simulink library "myLibrary"  (R2017b)
settings: Solver=VariableStepAuto  StartTime=0.0  StopTime=10.0  RelTol=1e-3
undefined symbols (not defined in the file): p, windData
libraries: aerolibwind2 x7, lowLevel x4, myLibrary x3, simulink x2, aerolibwindfilters x1, sharedtransform x1
settings Model: Creator=M.Cobb  LastModifiedBy=M.Cobb
settings CodeAppCC: StateflowObjectComments=on

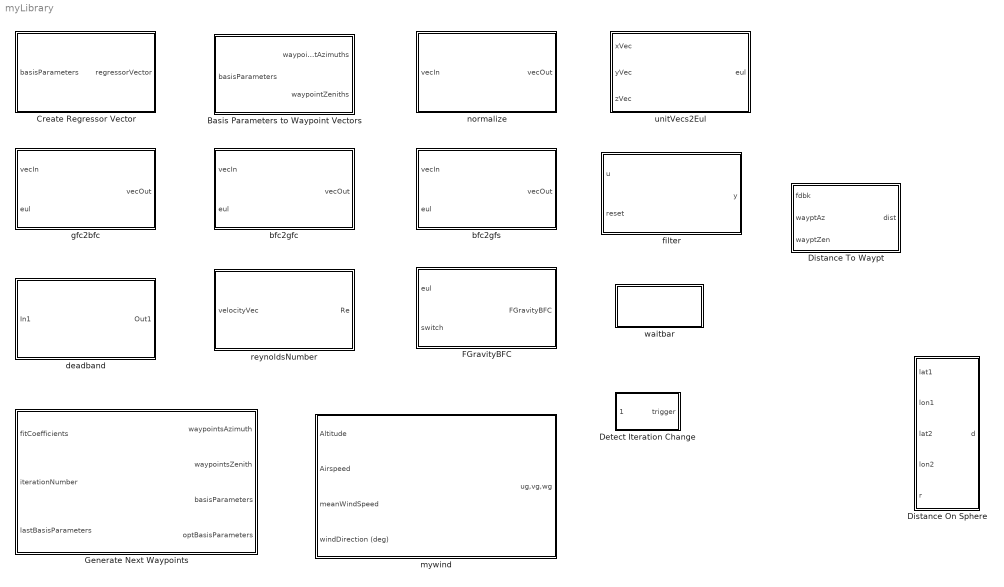
== system myLibrary ==
  Basis Parameters to Waypoint Vectors : Subsystem
  Create Regressor Vector : Subsystem
  Detect Iteration Change : Subsystem
  Distance On Sphere : Subsystem
  Distance To Waypt : Subsystem
  FGravityBFC : Subsystem
  Generate Next Waypoints : Subsystem
  bfc2gfc : Subsystem
  bfc2gfs : Subsystem
  deadband : Subsystem
  filter : Subsystem
  gfc2bfc : Subsystem
  mywind : Subsystem  mask(Wind Turbulence Model){units=Metric (MKS), spec=MIL-F-8785C, model=Continuous Von Karman (+q +r), Wdeg=0, TurbProb=10^-2 - Light, L_high=762, Wingspan=p.wingSpan, ts=p.Ts, Seed=[23341 23342 23343 23344], T_on=on}
      mask prompts: units "aeroblks:aeroblkwind:blockWindTurbulenceModelParamUnits"; spec "aeroblks:aeroblkwind:blockWindTurbulenceModelParamSpecification"; model "aeroblks:aeroblkwind:blockWindTurbulenceModelParamModeltype"; Wdeg "Wind direction at 6 m (degrees clockwise from north):"; TurbProb "aeroblks:aeroblkwind:blockWindTurbulenceModelParamProbabilityofexceedanceofhighaltitudeintensity"; L_high "Scale length at medium/high altitudes (m):"; Wingspan "Wingspan (m):"; ts "Band limited noise sample time (sec):"; Seed "Band limited noise sample time (sec):"; T_on "aeroblks:aeroblkwind:blockWindTurbulenceModelParamTurbulenceon"
      mask help: aeroblks:aeroblkwind:blockWindTurbulenceModelDesc
      mask init:
      | % index = strfind(model,' ');
      | % disp1 = model(1:index(1)-1);
      | % disp2 = model(index(1)+1:index(end-1)-1);
      | % disp3 = model(index(end-1)+1:end);
      | % 
      | h_vec = [.5 1.75 3.75 7.5 15 25 35 45 55 65 75 80]*1000;% feet
      | sigma_vec(1,:) = [3.2 2.2 1.5 zeros(1,9)]; % ft/sec
      | sigma_vec(2,:) = [4.2 3.6 3.3 1.6 zeros(1,8)];
      | sigma_vec(3,:) = [6.6 6.9 7.4 6.7 4.6 2.7 0.4 zeros(1,5)];
      | sigma_vec(4,:) = [8.6 9.6 10.6 10.1 8.0 6.6 5.0 4.2 2.7 zeros(1,3)];
      | sigma_vec(5,:) = [11.8 13.0 16.0 15.1 11.6 9.7 8.1 8.2 7.9 4.9 3.2 2.1];
      | sigma_vec(6,:) = [15.6 17.6 23.0 23.6 22.1 20.0 16.0 15.1 12.1 7.9 6.2 5.1];
      | sigma_vec(7,:) = [18.7 21.5 28.4 30.2 30.7 31.0 25.2 23.1 17.5 10.7 8.4 7.2];
      | max_height_low = 1000;
      | if strcmp(spec,'MIL-F-8785C')
      |     min_height_high = 2000;
      | else
      | 	min_height_high = 1750;
      | end
      | % [ports] = aeroicon('aeroblkwindturb2','icon');
      | % 
      | % dt=ts;
      mask Help: eval('asbhelp(''Von Karman Wind Turbulence Model (Continuous)'')');
      mask TypeOptions units: aeroblks:aeroblkwind:blockWindTurbulenceModelParamComboMetricMKS | aeroblks:aeroblkwind:blockWindTurbulenceModelParamComboEnglishVelocityinfts | aeroblks:aeroblkwind:blockWindTurbulenceModelParamComboEnglishVelocityinkts
      mask TypeOptions spec: aeroblks:aeroblkwind:blockWindTurbulenceModelParamComboMILF8785C | aeroblks:aeroblkwind:blockWindTurbulenceModelParamComboMILHDBK1797 | aeroblks:aeroblkwind:blockWindTurbulenceModelParamComboMILHDBK1797B
      mask TypeOptions model: aeroblks:aeroblkwind:blockWindTurbulenceModelParamComboContinuousVonKarmanqr1 | aeroblks:aeroblkwind:blockWindTurbulenceModelParamComboContinuousVonKarmanqr2 | aeroblks:aeroblkwind:blockWindTurbulenceModelParamComboContinuousVonKarmanqr3 | aeroblks:aeroblkwind:blockWindTurbulenceModelParamComboContinuousDrydenqr1 | aeroblks:aeroblkwind:blockWindTurbulenceModelParamComboContinuousDrydenqr2 | aeroblks:aeroblkwind:blockWindTurbulenceModelParamComboContinuousDrydenqr3 | aeroblks:aeroblkwind:blockWindTurbulenceModelParamComboDiscreteDrydenqr1 | aeroblks:aeroblkwind:blockWindTurbulenceModelParamComboDiscreteDrydenqr2 | aeroblks:aeroblkwind:blockWindTurbulenceModelParamComboDiscreteDrydenqr3
      mask Callback model: aeroicon('aeroblkwindturb2');
      mask TypeOptions TurbProb: aeroblks:aeroblkwind:blockWindTurbulenceModelParamCombo2x101 | aeroblks:aeroblkwind:blockWindTurbulenceModelParamCombo101 | aeroblks:aeroblkwind:blockWindTurbulenceModelParamCombo102Light | aeroblks:aeroblkwind:blockWindTurbulenceModelParamCombo103Moderate | aeroblks:aeroblkwind:blockWindTurbulenceModelParamCombo104 | aeroblks:aeroblkwind:blockWindTurbulenceModelParamCombo105Severe | aeroblks:aeroblkwind:blockWindTurbulenceModelParamCombo106
      mask Display:
      | port_label('output',1,'vWind','texmode','on');
      | port_label('input',1,'altitude (m)','texmode','on');
      | port_label('input',2,'airspeed (m/s)','texmode','on');
      | port_label('input',3,'meanWindSpeed (m/s)','texmode','on');
      | port_label('input',4,'wind direction (deg)','texmode','on');
      | % port_label(ports(5).type,ports(5).port,ports(5).txt,'texmode','on');
      | % [x y highstr lowstr maxy miny] = aeroimage('wind',gcbh,[disp2 '\n' disp3],disp1);
      | % plot(x,y)
      | % text(0.5,miny-0.05,lowstr,'HorizontalAlignment','center','verticalalignment','top')
      | % text(0.5,maxy,highstr,'HorizontalAlignment','center','verticalalignment','bottom')
  normalize : Subsystem
  reynoldsNumber : Subsystem
  unitVecs2Eul : Subsystem
  waitbar : Subsystem

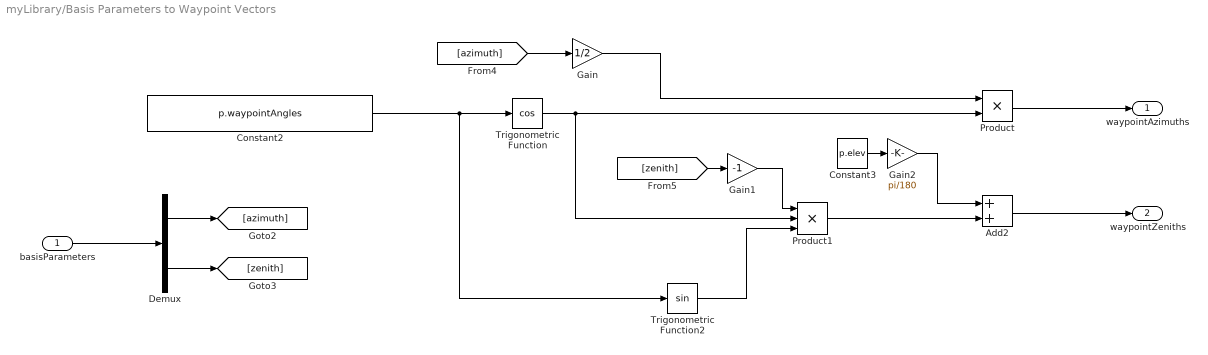
== system myLibrary/Basis Parameters to Waypoint Vectors ==
  basisParameters : Inport
  Add2 : Sum
  Constant2 : Constant  Value=p.waypointAngles  SampleTime=-1
  Constant3 : Constant  Value=p.elev
  Demux : Demux  Outputs=2
  Gain : Gain  Gain=1/2
  Gain1 : Gain  Gain=-1
  Gain2 : Gain  Gain=pi/180
  Product : Product
  Product1 : Product  Inputs=3
  Trigonometric Function : Trigonometry  Operator=cos
  Trigonometric Function2 : Trigonometry
  waypointAzimuths : Outport
  waypointZeniths : Outport  Port=2
  wires:
  Gain/1 -> Product/1
  Product1/1 -> Add2/2
  Trigonometric Function2/1 -> Product1/3
  [azimuth] -> Gain/1
  Constant2/1 -> Trigonometric Function2/1, Trigonometric Function/1
  basisParameters/1 -> Demux/1
  Demux/1 -> [azimuth]
  [zenith] -> Gain1/1
  Gain1/1 -> Product1/1
  Demux/2 -> [zenith]
  Trigonometric Function/1 -> Product1/2, Product/2
  Constant3/1 -> Gain2/1
  Product/1 -> waypointAzimuths/1
  Add2/1 -> waypointZeniths/1
  Gain2/1 -> Add2/1

== system myLibrary/Create Regressor Vector ==
  basisParameters : Inport  PortDimensions=2
  Constant2 : Constant
  Demux : Demux  Outputs=2
  Mux : Mux  Inputs=5
  Product : Product
  Product1 : Product
  regressorVector : Outport  PortDimensions=5
  wires:
  Demux/2 -> Product/2, Product/1, Mux/4
  Demux/1 -> Product1/2, Product1/1, Mux/2
  Mux/1 -> regressorVector/1
  Product/1 -> Mux/5
  Constant2/1 -> Mux/1
  Product1/1 -> Mux/3
  basisParameters/1 -> Demux/1

== system myLibrary/Detect Iteration Change ==
  wyptIdx : Inport
  Add1 : Sum  Inputs=+-
  Compare To Constant : simulink/Logic and Bit Operations/Compare To Constant  relop===  const=-p.num  OutDataTypeStr=boolean
  Delay1 : Delay  DelayLength=1  InitialCondition=0
  trigger : Outport
  wires:
  Add1/1 -> Compare To Constant/1
  wyptIdx/1 -> Delay1/1, Add1/1
  Compare To Constant/1 -> trigger/1
  Delay1/1 -> Add1/2

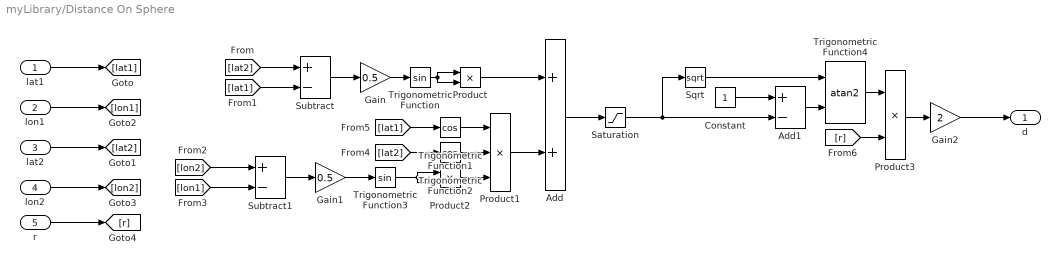
== system myLibrary/Distance On Sphere ==
  lat1 : Inport
  lon1 : Inport  Port=2
  lat2 : Inport  Port=3
  lon2 : Inport  Port=4
  r : Inport  Port=5
  Add : Sum
  Add1 : Sum  Inputs=+-
  Constant : Constant
  Gain : Gain  Gain=0.5
  Gain1 : Gain  Gain=0.5
  Gain2 : Gain  Gain=2
  Product : Product
  Product1 : Product  Inputs=3
  Product2 : Product
  Product3 : Product
  Saturation : Saturate  UpperLimit=1  LowerLimit=0
  Sqrt : Sqrt  SaturateOnIntegerOverflow=on
  Subtract : Sum  Inputs=+-
  Subtract1 : Sum  Inputs=+-
  Trigonometric Function : Trigonometry
  Trigonometric Function1 : Trigonometry  Operator=cos
  Trigonometric Function2 : Trigonometry  Operator=cos
  Trigonometric Function3 : Trigonometry
  Trigonometric Function4 : Trigonometry  Operator=atan2
  d : Outport
  wires:
  Gain/1 -> Trigonometric Function/1
  Subtract/1 -> Gain/1
  Trigonometric Function/1 -> Product/2, Product/1
  Subtract1/1 -> Gain1/1
  [lon1] -> Subtract1/2
  [lon2] -> Subtract1/1
  Sqrt/1 -> Trigonometric Function4/1
  Trigonometric Function1/1 -> Product1/1
  Trigonometric Function4/1 -> Product3/1
  Product/1 -> Add/1
  [r] -> Product3/2
  Constant/1 -> Add1/1
  [lat1] -> Subtract/2
  Product1/1 -> Add/2
  Trigonometric Function2/1 -> Product1/2
  Add/1 -> Saturation/1
  Add1/1 -> Trigonometric Function4/2
  Product3/1 -> Gain2/1
  [lat1] -> Trigonometric Function1/1
  [lat2] -> Trigonometric Function2/1
  Product2/1 -> Product1/3
  [lat2] -> Subtract/1
  Saturation/1 -> Add1/2, Sqrt/1
  Trigonometric Function3/1 -> Product2/2, Product2/1
  Gain2/1 -> d/1
  Gain1/1 -> Trigonometric Function3/1
  lon1/1 -> [lon1]
  lat1/1 -> [lat1]
  lat2/1 -> [lat2]
  lon2/1 -> [lon2]
  r/1 -> [r]

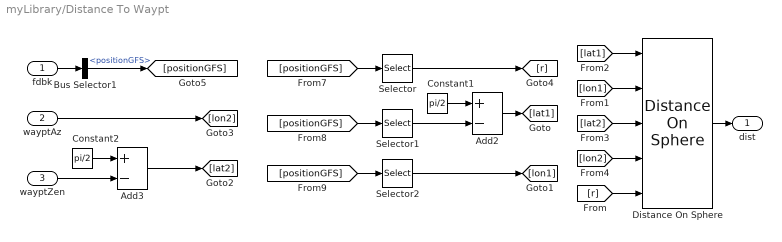
== system myLibrary/Distance To Waypt ==
  fdbk : Inport
  wayptAz : Inport  Port=2
  wayptZen : Inport  Port=3
  Add2 : Sum  Inputs=+-
  Add3 : Sum  Inputs=+-
  Bus Selector1 : BusSelector  OutputSignals=positionGFS
  Constant1 : Constant  Value=pi/2
  Constant2 : Constant  Value=pi/2
  Distance On Sphere : myLibrary/Distance On Sphere
  Selector : Selector  InputPortWidth=3  IndexOptions=Index vector (dialog)  Indices=1  OutputSizes=1
  Selector1 : Selector  InputPortWidth=3  IndexOptions=Index vector (dialog)  Indices=3  OutputSizes=1
  Selector2 : Selector  InputPortWidth=3  IndexOptions=Index vector (dialog)  Indices=2  OutputSizes=1
  dist : Outport
  wires:
  fdbk/1 -> Bus Selector1/1
  Bus Selector1/1 -> [positionGFS]  "<positionGFS>"
  [positionGFS] -> Selector/1
  Selector/1 -> [r]
  [positionGFS] -> Selector1/1
  Constant1/1 -> Add2/1
  Add2/1 -> [lat1]
  Selector1/1 -> Add2/2
  [positionGFS] -> Selector2/1
  Selector2/1 -> [lon1]
  Constant2/1 -> Add3/1
  wayptZen/1 -> Add3/2
  Add3/1 -> [lat2]
  wayptAz/1 -> [lon2]
  Distance On Sphere/1 -> dist/1
  [r] -> Distance On Sphere/5
  [lon1] -> Distance On Sphere/2
  [lat1] -> Distance On Sphere/1
  [lat2] -> Distance On Sphere/3
  [lon2] -> Distance On Sphere/4

== system myLibrary/FGravityBFC ==
  eul : Inport
  switch : Inport  Port=2
  Constant : Constant  Value=[0 0 -p.g*p.mass]'
  Constant1 : Constant  Value=[0 0 0]
  Product : Product  Multiplication=Matrix(*)
  Product1 : Product  Inputs=/  Multiplication=Matrix(*)
  Switch : Switch  Criteria=u2 ~= 0
  eul2rot : lowLevel/eul2rot
  FGravityBFC : Outport
  wires:
  eul2rot/1 -> Product1/1
  eul/1 -> eul2rot/1
  Constant1/1 -> Switch/3
  switch/1 -> Switch/2
  Product/1 -> Switch/1
  Switch/1 -> FGravityBFC/1
  Product1/1 -> Product/1
  Constant/1 -> Product/2

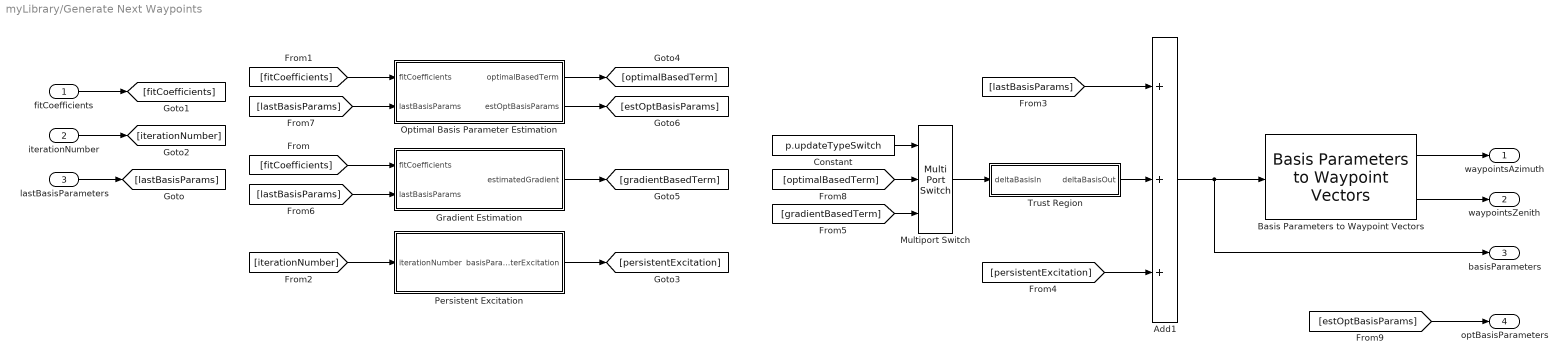
== system myLibrary/Generate Next Waypoints ==
  fitCoefficients : Inport  PortDimensions=5
  iterationNumber : Inport  Port=2
  lastBasisParameters : Inport  Port=3
  Add1 : Sum  Inputs=+++
  Basis Parameters to Waypoint Vectors : myLibrary/Basis Parameters to Waypoint Vectors
  Constant : Constant  Value=p.updateTypeSwitch
  Gradient Estimation : Subsystem
  Multiport Switch : MultiPortSwitch  Inputs=2
  Optimal Basis Parameter Estimation : Subsystem
  Persistent Excitation : Subsystem
  Trust Region : Subsystem
  waypointsAzimuth : Outport
  waypointsZenith : Outport  Port=2
  basisParameters : Outport  Port=3
  optBasisParameters : Outport  Port=4
  wires:
  [persistentExcitation] -> Add1/3
  Trust Region/1(deltaBasisOut) -> Add1/2
  [lastBasisParams] -> Add1/1
  Constant/1 -> Multiport Switch/1
  [gradientBasedTerm] -> Multiport Switch/3
  [optimalBasedTerm] -> Multiport Switch/2
  [estOptBasisParams] -> optBasisParameters/1
  Optimal Basis Parameter Estimation/2(estOptBasisParams) -> [estOptBasisParams]
  [lastBasisParams] -> Optimal Basis Parameter Estimation/2(lastBasisParams)
  [lastBasisParams] -> Gradient Estimation/2(lastBasisParams)
  Optimal Basis Parameter Estimation/1(optimalBasedTerm) -> [optimalBasedTerm]
  Gradient Estimation/1(estimatedGradient) -> [gradientBasedTerm]
  Persistent Excitation/1(basisParameterExcitation) -> [persistentExcitation]
  [iterationNumber] -> Persistent Excitation/1(iterationNumber)
  iterationNumber/1 -> [iterationNumber]
  [fitCoefficients] -> Optimal Basis Parameter Estimation/1(fitCoefficients)
  [fitCoefficients] -> Gradient Estimation/1(fitCoefficients)
  fitCoefficients/1 -> [fitCoefficients]
  lastBasisParameters/1 -> [lastBasisParams]
  Multiport Switch/1 -> Trust Region/1(deltaBasisIn)
  Basis Parameters to Waypoint Vectors/2 -> waypointsZenith/1
  Basis Parameters to Waypoint Vectors/1 -> waypointsAzimuth/1
  Add1/1 -> basisParameters/1, Basis Parameters to Waypoint Vectors/1

== system myLibrary/bfc2gfc ==
  vecIn : Inport
  eul : Inport  Port=2
  Product : Product  Multiplication=Matrix(*)
  eul2rot : lowLevel/eul2rot
  vecOut : Outport
  wires:
  eul/1 -> eul2rot/1
  Product/1 -> vecOut/1
  eul2rot/1 -> Product/1
  vecIn/1 -> Product/2

== system myLibrary/bfc2gfs ==
  vecIn : Inport
  eul : Inport  Port=2
  bfc2gfc : myLibrary/bfc2gfc
  crtPos2sphPos : lowLevel/crtPos2sphPos
  vecOut : Outport
  wires:
  vecIn/1 -> bfc2gfc/1
  eul/1 -> bfc2gfc/2
  bfc2gfc/1 -> crtPos2sphPos/1
  crtPos2sphPos/1 -> vecOut/1

== system myLibrary/deadband ==
  In1 : Inport
  Abs : Abs
  Constant : Constant  Value=1e-10
  Constant1 : Constant  Value=0
  Subtract : Sum  Inputs=+-
  Switch : Switch  Criteria=u2 > Threshold
  Out1 : Outport
  wires:
  In1/1 -> Switch/1, Abs/1
  Abs/1 -> Subtract/1
  Subtract/1 -> Switch/2
  Constant/1 -> Subtract/2
  Constant1/1 -> Switch/3
  Switch/1 -> Out1/1

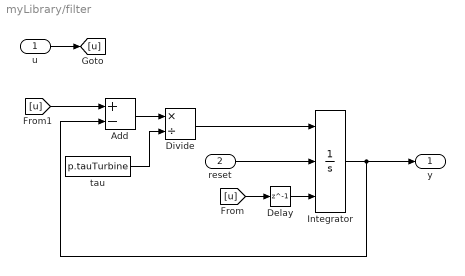
== system myLibrary/filter ==
  u : Inport
  reset : Inport  Port=2
  Add : Sum  Inputs=+-
  Delay : Delay  DelayLength=1  InitialCondition=windData.altitude146.data(1)
  Divide : Product  Inputs=*/
  Integrator : Integrator  ExternalReset=rising  InitialConditionSource=external
  tau : Constant  Value=p.tauTurbine
  y : Outport
  wires:
  Add/1 -> Divide/1
  Divide/1 -> Integrator/1
  Integrator/1 -> y/1, Add/2
  reset/1 -> Integrator/2
  tau/1 -> Divide/2
  Delay/1 -> Integrator/3
  u/1 -> [u]
  [u] -> Delay/1
  [u] -> Add/1

== system myLibrary/gfc2bfc ==
  vecIn : Inport
  eul : Inport  Port=2
  Product : Product  Multiplication=Matrix(*)
  Product1 : Product  Inputs=/  Multiplication=Matrix(*)
  eul2rot : lowLevel/eul2rot
  vecOut : Outport
  wires:
  Product1/1 -> Product/1
  eul2rot/1 -> Product1/1
  eul/1 -> eul2rot/1
  vecIn/1 -> Product/2
  Product/1 -> vecOut/1

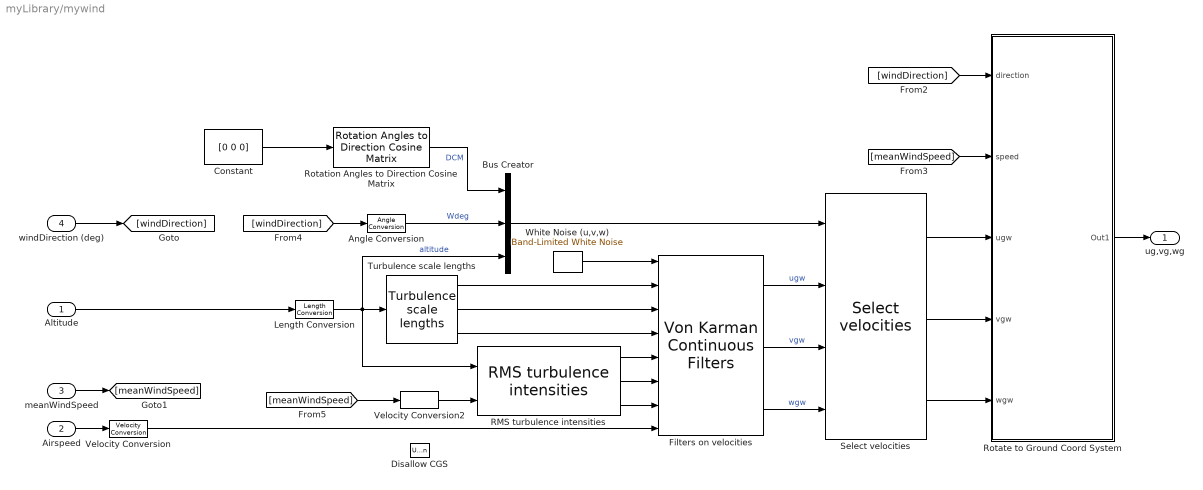
== system myLibrary/mywind ==
  Altitude : Inport  Unit=m
  Airspeed : Inport  Port=2  Unit=m/s
  meanWindSpeed : Inport  Port=3  Unit=m/s
  windDirection (deg) : Inport  Port=4  Unit=deg
  Angle Conversion : aerolibwind2/Dryden Wind Turbulence Model  (Continuous (+q -r))/Angle Conversion
      settings: SourceProductName=Aerospace Blockset  SourceProductBaseCode=AE
  Bus Creator : BusCreator  Inputs=3
  Constant : Constant  Value=[0 0 0]
  Disallow CGS : UnitConfiguration  UnitSystemsStr=English,SI,SI (extended)  AllowAllUnitSystems=off
  Filters on velocities : aerolibwindfilters/Von Karman Continuous Filters  SystemSampleTime=-1
      settings: SourceProductName=Aerospace Blockset  SourceProductBaseCode=AE
  Length Conversion : aerolibwind2/Dryden Wind Turbulence Model  (Continuous (+q -r))/Length Conversion
      settings: SourceProductName=Aerospace Blockset  SourceProductBaseCode=AE
  RMS turbulence intensities : aerolibwind2/Dryden Wind Turbulence Model  (Continuous (+q -r))/RMS turbulence  intensities
      settings: SourceProductName=Aerospace Blockset  SourceProductBaseCode=AE
  Rotate to Ground Coord System : Subsystem
  Rotation Angles to Direction Cosine Matrix : sharedtransform/Rotation Angles to Direction Cosine Matrix  rotationOrder=ZYX
      settings: SourceProductBaseCode=AE
  Select velocities : aerolibwind2/Dryden Wind Turbulence Model  (Continuous (+q -r))/Select velocities
      settings: SourceProductName=Aerospace Blockset  SourceProductBaseCode=AE
  Turbulence scale lengths : aerolibwind2/Dryden Wind Turbulence Model  (Continuous (+q -r))/Turbulence scale lengths
      settings: SourceProductName=Aerospace Blockset  SourceProductBaseCode=AE
  Velocity Conversion : aerolibwind2/Dryden Wind Turbulence Model  (Continuous (+q -r))/Velocity Conversion
      settings: SourceProductName=Aerospace Blockset  SourceProductBaseCode=AE
  Velocity Conversion2 : aerolibwind2/Dryden Wind Turbulence Model  (Continuous (+q -r))/Velocity Conversion2
      settings: SourceProductName=Aerospace Blockset  SourceProductBaseCode=AE
  White Noise (u,v,w) : simulink/Sources/Band-Limited White Noise  Cov=[1 1 1]*pi  Ts=ts  seed=Seed(1:3)
  ug,vg,wg : Outport  Unit=m/s
  wires:
  Velocity Conversion/1 -> Filters on velocities/8
  White Noise (u,v,w)/1 -> Filters on velocities/1
  Filters on velocities/3 -> Select velocities/4  "wgw"
  Bus Creator/1 -> Select velocities/1
  Altitude/1 -> Length Conversion/1
  Angle Conversion/1 -> Bus Creator/2  "Wdeg"
  Turbulence scale lengths/3 -> Filters on velocities/4
  Turbulence scale lengths/1 -> Filters on velocities/2
  Filters on velocities/1 -> Select velocities/2  "ugw"
  Rotation Angles to Direction Cosine Matrix/1 -> Bus Creator/1  "DCM"
  Airspeed/1 -> Velocity Conversion/1
  RMS turbulence intensities/3 -> Filters on velocities/7
  RMS turbulence intensities/2 -> Filters on velocities/6
  Velocity Conversion2/1 -> RMS turbulence intensities/2
  Length Conversion/1 -> Turbulence scale lengths/1, RMS turbulence intensities/1, Bus Creator/3  "altitude"
  RMS turbulence intensities/1 -> Filters on velocities/5
  Filters on velocities/2 -> Select velocities/3  "vgw"
  Turbulence scale lengths/2 -> Filters on velocities/3
  windDirection (deg)/1 -> [windDirection]
  meanWindSpeed/1 -> [meanWindSpeed]
  [windDirection] -> Angle Conversion/1
  [meanWindSpeed] -> Velocity Conversion2/1
  [windDirection] -> Rotate to Ground Coord System/1(direction)
  [meanWindSpeed] -> Rotate to Ground Coord System/2(speed)
  Select velocities/1 -> Rotate to Ground Coord System/3(ugw)
  Select velocities/2 -> Rotate to Ground Coord System/4(vgw)
  Select velocities/3 -> Rotate to Ground Coord System/5(wgw)
  Rotate to Ground Coord System/1(Out1) -> ug,vg,wg/1
  Constant/1 -> Rotation Angles to Direction Cosine Matrix/1

== system myLibrary/normalize ==
  vecIn : Inport
  Divide : Product  Inputs=*/
  Dot Product : DotProduct  InputSameDT=on  OutDataTypeStr=Inherit: Inherit via internal rule
  Sqrt : Sqrt  SaturateOnIntegerOverflow=on
  vecOut : Outport
  wires:
  vecIn/1 -> Divide/1, Dot Product/2, Dot Product/1
  Dot Product/1 -> Sqrt/1
  Sqrt/1 -> Divide/2
  Divide/1 -> vecOut/1

== system myLibrary/reynoldsNumber ==
  velocityVec : Inport
  Dot Product : DotProduct  InputSameDT=on  OutDataTypeStr=Inherit: Inherit via internal rule
  Gain : Gain  Gain=(p.rho*p.refLengthWing)/p.viscosity
  Sqrt : Sqrt  SaturateOnIntegerOverflow=on
  Re : Outport
  wires:
  Gain/1 -> Re/1
  velocityVec/1 -> Dot Product/2, Dot Product/1
  Dot Product/1 -> Sqrt/1
  Sqrt/1 -> Gain/1

== system myLibrary/unitVecs2Eul ==
  xVec : Inport
  yVec : Inport  Port=2
  zVec : Inport  Port=3
  unitVecs2Eul : MATLAB Function  TreatAsAtomicUnit=on
  eul : Outport
  wires:
  xVec/1 -> unitVecs2Eul/1(xVec)
  yVec/1 -> unitVecs2Eul/2(yVec)
  zVec/1 -> unitVecs2Eul/3(zVec)
  unitVecs2Eul/1(eul) -> eul/1

== system myLibrary/waitbar ==
  Clock : Clock
  Constant : Constant  Value=p.T
  Embedded MATLAB Function : MATLAB Function  TreatAsAtomicUnit=on
  Scope : Scope
  wires:
  Embedded MATLAB Function/1(y) -> Scope/1
  Constant/1 -> Embedded MATLAB Function/2(u2)
  Clock/1 -> Embedded MATLAB Function/1(u1)

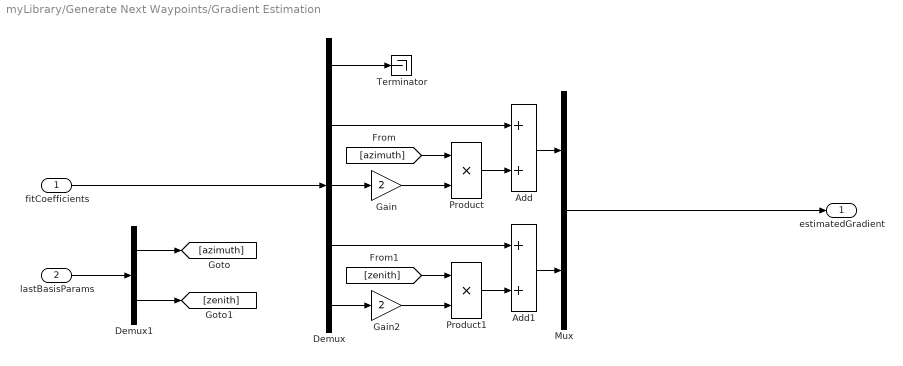
== system myLibrary/Generate Next Waypoints/Gradient Estimation ==
  fitCoefficients : Inport  PortDimensions=5
  lastBasisParams : Inport  Port=2  PortDimensions=2
  Add : Sum
  Add1 : Sum
  Demux : Demux  Outputs=5
  Demux1 : Demux  Outputs=2
  Gain : Gain  Gain=2
  Gain2 : Gain  Gain=2
  Mux : Mux  Inputs=2
  Product : Product
  Product1 : Product
  Terminator : Terminator
  estimatedGradient : Outport
  wires:
  Demux/4 -> Add1/1
  Demux/5 -> Gain2/1
  [zenith] -> Product1/1
  Gain2/1 -> Product1/2
  Add1/1 -> Mux/2
  Product1/1 -> Add1/2
  Gain/1 -> Product/2
  [azimuth] -> Product/1
  Product/1 -> Add/2
  Demux1/2 -> [zenith]
  Demux1/1 -> [azimuth]
  lastBasisParams/1 -> Demux1/1
  Demux/3 -> Gain/1
  Demux/2 -> Add/1
  Add/1 -> Mux/1
  Demux/1 -> Terminator/1
  Mux/1 -> estimatedGradient/1
  fitCoefficients/1 -> Demux/1

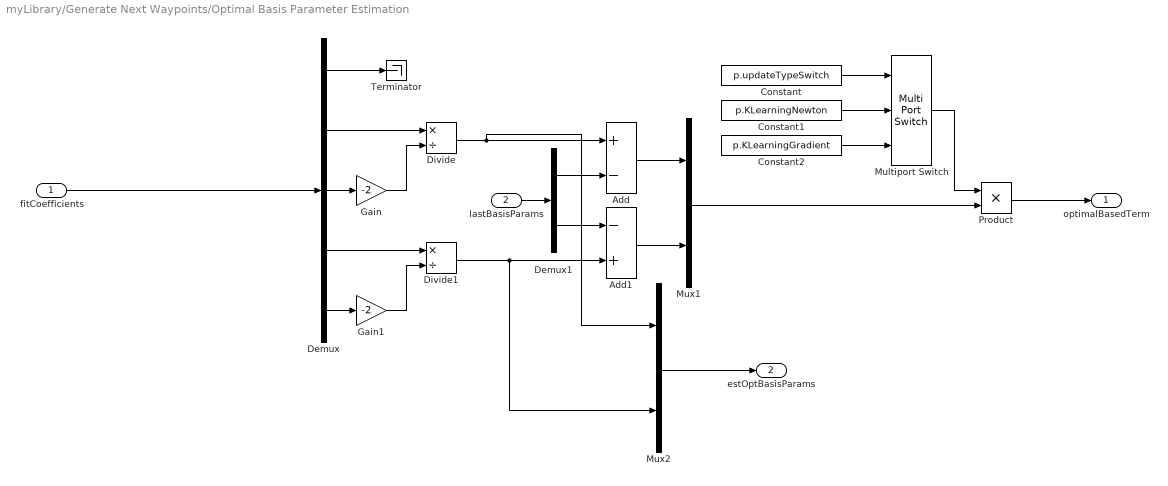
== system myLibrary/Generate Next Waypoints/Optimal Basis Parameter Estimation ==
  fitCoefficients : Inport  PortDimensions=5
  lastBasisParams : Inport  Port=2  PortDimensions=2
  Add : Sum  Inputs=+-
  Add1 : Sum  Inputs=-+
  Constant : Constant  Value=p.updateTypeSwitch
  Constant1 : Constant  Value=p.KLearningNewton
  Constant2 : Constant  Value=p.KLearningGradient
  Demux : Demux  Outputs=5
  Demux1 : Demux  Outputs=2
  Divide : Product  Inputs=*/
  Divide1 : Product  Inputs=*/
  Gain : Gain  Gain=-2
  Gain1 : Gain  Gain=-2
  Multiport Switch : MultiPortSwitch  Inputs=2
  Mux1 : Mux  Inputs=2
  Mux2 : Mux  Inputs=2
  Product : Product
  Terminator : Terminator
  optimalBasedTerm : Outport
  estOptBasisParams : Outport  Port=2
  wires:
  Mux2/1 -> estOptBasisParams/1
  Add/1 -> Mux1/1
  Add1/1 -> Mux1/2
  Divide1/1 -> Add1/2, Mux2/2
  Divide/1 -> Add/1, Mux2/1
  Demux1/2 -> Add1/1
  Demux1/1 -> Add/2
  lastBasisParams/1 -> Demux1/1
  Demux/2 -> Divide/1
  Demux/1 -> Terminator/1
  Demux/3 -> Gain/1
  Gain1/1 -> Divide1/2
  Gain/1 -> Divide/2
  Demux/4 -> Divide1/1
  fitCoefficients/1 -> Demux/1
  Demux/5 -> Gain1/1
  Multiport Switch/1 -> Product/1
  Product/1 -> optimalBasedTerm/1
  Mux1/1 -> Product/2
  Constant/1 -> Multiport Switch/1
  Constant2/1 -> Multiport Switch/3
  Constant1/1 -> Multiport Switch/2

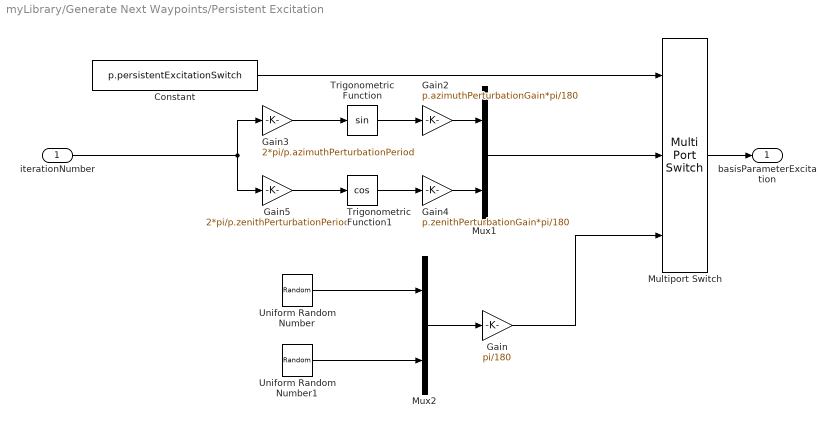
== system myLibrary/Generate Next Waypoints/Persistent Excitation ==
  iterationNumber : Inport
  Constant : Constant  Value=p.persistentExcitationSwitch
  Gain : Gain  Gain=pi/180
  Gain2 : Gain  Gain=p.azimuthPerturbationGain*pi/180
  Gain3 : Gain  Gain=2*pi/p.azimuthPerturbationPeriod
  Gain4 : Gain  Gain=p.zenithPerturbationGain*pi/180
  Gain5 : Gain  Gain=2*pi/p.zenithPerturbationPeriod
  Multiport Switch : MultiPortSwitch  Inputs=2
  Mux1 : Mux  Inputs=2
  Mux2 : Mux  Inputs=2
  Trigonometric Function : Trigonometry
  Trigonometric Function1 : Trigonometry  Operator=cos
  Uniform Random Number : UniformRandomNumber  Minimum=-p.azimuthPerturbationGain  Maximum=p.azimuthPerturbationGain  Seed=92881
  Uniform Random Number1 : UniformRandomNumber  Minimum=-p.zenithPerturbationGain  Maximum=p.zenithPerturbationGain  Seed=52787
  basisParameterExcitation : Outport
  wires:
  Gain/1 -> Multiport Switch/3
  Uniform Random Number1/1 -> Mux2/2
  Uniform Random Number/1 -> Mux2/1
  Mux2/1 -> Gain/1
  Mux1/1 -> Multiport Switch/2
  Constant/1 -> Multiport Switch/1
  Multiport Switch/1 -> basisParameterExcitation/1
  iterationNumber/1 -> Gain3/1, Gain5/1
  Gain4/1 -> Mux1/2
  Gain5/1 -> Trigonometric Function1/1
  Trigonometric Function/1 -> Gain2/1
  Trigonometric Function1/1 -> Gain4/1
  Gain2/1 -> Mux1/1
  Gain3/1 -> Trigonometric Function/1

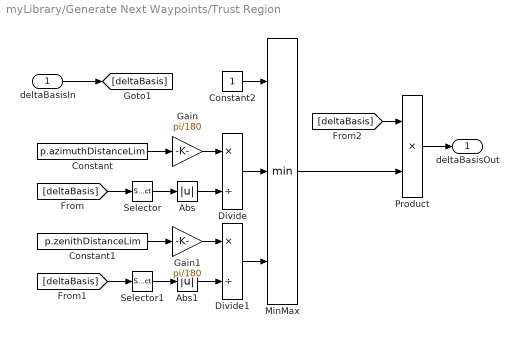
== system myLibrary/Generate Next Waypoints/Trust Region ==
  deltaBasisIn : Inport
  Abs : Abs
  Abs1 : Abs
  Constant : Constant  Value=p.azimuthDistanceLim
  Constant1 : Constant  Value=p.zenithDistanceLim
  Constant2 : Constant
  Divide : Product  Inputs=*/
  Divide1 : Product  Inputs=*/
  Gain : Gain  Gain=pi/180
  Gain1 : Gain  Gain=pi/180
  MinMax : MinMax  Inputs=3
  Product : Product
  Selector : Selector  InputPortWidth=2  IndexOptions=Index vector (dialog)  Indices=1  OutputSizes=1
  Selector1 : Selector  InputPortWidth=2  IndexOptions=Index vector (dialog)  Indices=2  OutputSizes=1
  deltaBasisOut : Outport
  wires:
  deltaBasisIn/1 -> [deltaBasis]
  Product/1 -> deltaBasisOut/1
  MinMax/1 -> Product/2
  [deltaBasis] -> Product/1
  Constant2/1 -> MinMax/1
  Constant1/1 -> Gain1/1
  [deltaBasis] -> Selector1/1
  Selector1/1 -> Abs1/1
  Selector/1 -> Abs/1
  Divide1/1 -> MinMax/3
  Abs/1 -> Divide/2
  Divide/1 -> MinMax/2
  Constant/1 -> Gain/1
  [deltaBasis] -> Selector/1
  Abs1/1 -> Divide1/2
  Gain/1 -> Divide/1
  Gain1/1 -> Divide1/1

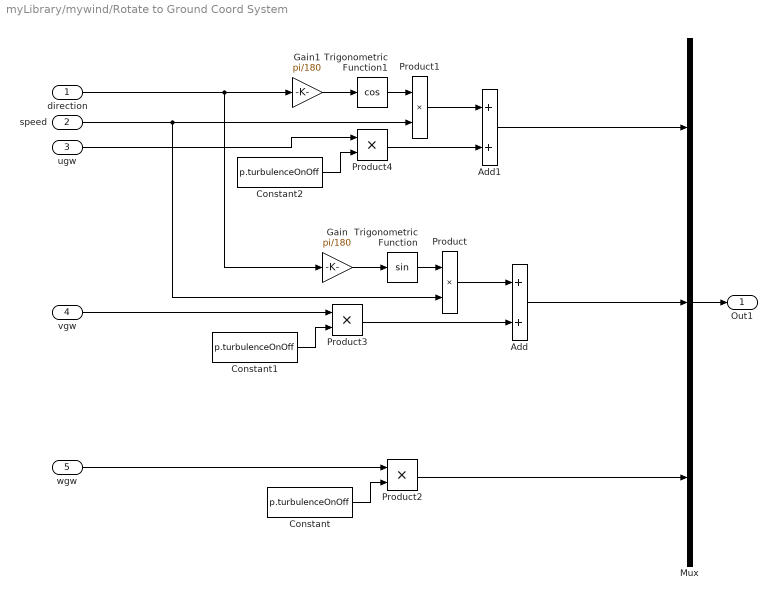
== system myLibrary/mywind/Rotate to Ground Coord System ==
  direction : Inport
  speed : Inport  Port=2
  ugw : Inport  Port=3
  vgw : Inport  Port=4
  wgw : Inport  Port=5
  Add : Sum
  Add1 : Sum
  Constant : Constant  Value=p.turbulenceOnOff
  Constant1 : Constant  Value=p.turbulenceOnOff
  Constant2 : Constant  Value=p.turbulenceOnOff
  Gain : Gain  Gain=pi/180
  Gain1 : Gain  Gain=pi/180
  Mux : Mux  Inputs=3
  Product{,1..4} (5 alike) : Product
  Trigonometric Function : Trigonometry
  Trigonometric Function1 : Trigonometry  Operator=cos
  Out1 : Outport
  wires:
  ugw/1 -> Product4/1
  Product4/1 -> Add1/2
  Constant2/1 -> Product4/2
  vgw/1 -> Product3/1
  Product3/1 -> Add/2
  Constant1/1 -> Product3/2
  Product2/1 -> Mux/3
  wgw/1 -> Product2/1
  Constant/1 -> Product2/2
  Mux/1 -> Out1/1
  Trigonometric Function1/1 -> Product1/1
  Gain1/1 -> Trigonometric Function1/1
  Product/1 -> Add/1
  Add1/1 -> Mux/1
  Trigonometric Function/1 -> Product/1
  Product1/1 -> Add1/1
  Gain/1 -> Trigonometric Function/1
  direction/1 -> Gain/1, Gain1/1
  Add/1 -> Mux/2
  speed/1 -> Product1/2, Product/2

== matlab function myLibrary/waitbar/Embedded MATLAB Function ==
  settings: fimath=|
      | fimath(...
      | 'RoundMode', 'floor',...
      | 'OverflowMode', 'wrap',...
      | 'ProductMode', 'KeepLSB', 'ProductWordLength', 32,...
      | 'SumMode', 'KeepLSB', 'SumWordLength', 32,...
      | 'CastBeforeSum', false)
  data: u1 input; y output; u2 input
function y = fcn(u1, u2)
% This block supports an embeddable subset of the MATLAB language.
% See the help menu for details. 
coder.extrinsic('waitbar')
waitbar(u1/u2)
y = 1;

== matlab function myLibrary/unitVecs2Eul/unitVecs2Eul ==
  data: xVec input; eul output; yVec input; zVec input
function eul = unitVecs2Eul(xVec,yVec,zVec)
% Function to convert unit vectors to euler angles
R=[xVec(1) yVec(1) zVec(1);xVec(2) yVec(2) zVec(2);xVec(3) yVec(3) zVec(3)];
eul=rotm2eul(R,'ZYX');
end
